simulink model "AutoTransmission"  (R2020a)
settings: Solver=VariableStepAuto  StartTime=0.0  StopTime=10.0  RelTol=1e-3
PostLoadFcn:
  | NE_VEC=[799.9999999999999 1200 1600 2000 2400 2800 3200 3600 4000 4400 4800];
  | TH_VEC=[0;20;30;40;50;60;70;80;90;100];
  | EMAP=[-40 -44 -49 -53 -57 -61 -65 -70 -74 -78 -82;215 117 85 66 44 29 10 -2 -13 -22 -32;245 208 178 148 122 104 85 66 48 33 18;264 260 241 219 193 167 152 133 119 96 85;264 279 282 275 260 238 223 208 189 171 152;267 290 293 297 290 275 260 256 234 212 193;267 297 305 305 305 301 293 282 267 249 226;267 301 308 312 319 323 319 316 297 279 253;267 301 312 319 327 327 327 327 312 293 267;267 301 312 319 327 334 334 334 319 305 275];
  | Iei=0.0219914882835559;
  | CONVERTER_DATA=[0 137.4652089938063 2.232;0.1 137.065019156852 2.075;0.2 135.8644496459891 1.975;0.3 135.6643547275119 1.846;0.4 137.5652564530449 1.72;0.5 140.3665853117251 1.564;0.6 145.2689108144154 1.409;0.7 152.8725177165473 1.254;0.8 162.9773110996437 1.096;0.81 164.2779280697452 1.08;0.82 166.1788297952782 1.061;0.83 167.9796840615726 1.043;0.84 170.0806807055828 1.028;0.85 172.7819621050244 1.012;0.86 175.3831960452274 1.002;0.87 179.5851893332477 1.002;0.88 183.5870877027908 1.001;0.89 189.8900776348212 0.998;0.9 197.6937794554303 0.999;0.92 215.9024170368515 1.001;0.94 244.5159903790849 1.002];
undefined symbols (not defined in the file): Kfactor, speedratio, Torkratio
settings Model: Creator=Hp  LastModifiedBy=Hp

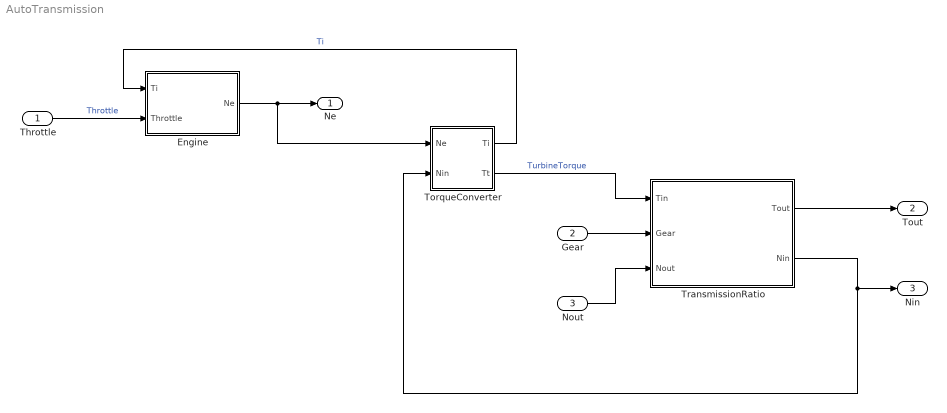
== system AutoTransmission ==
  Throttle : Inport
  Gear : Inport  Port=2
  Nout : Inport  Port=3
  Engine : Subsystem
  TorqueConverter : Subsystem
  TransmissionRatio : Subsystem
  Ne : Outport  Unit=rpm  VectorParamsAs1DForOutWhenUnconnected=off
  Tout : Outport  Port=2
  Nin : Outport  Port=3
  wires:
  TorqueConverter/1(Ti) -> Engine/1(Ti)  "Ti"
  Throttle/1 -> Engine/2(Throttle)  "Throttle"
  Engine/1(Ne) -> TorqueConverter/1(Ne), Ne/1
  TransmissionRatio/2(Nin) -> TorqueConverter/2(Nin), Nin/1
  TorqueConverter/2(Tt) -> TransmissionRatio/1(Tin)  "TurbineTorque"
  Gear/1 -> TransmissionRatio/2(Gear)
  Nout/1 -> TransmissionRatio/3(Nout)
  TransmissionRatio/1(Tout) -> Tout/1

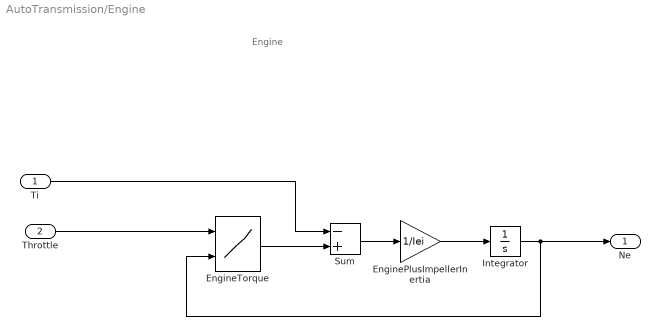
== system AutoTransmission/Engine ==
  note: Engine
  Ti : Inport
  Throttle : Inport  Port=2
  EnginePlusImpellerInertia : Gain  Gain=1/Iei  SaturateOnIntegerOverflow=on  OutDataTypeStr=Inherit: Same as input  ParamDataTypeStr=Inherit: Same as input
  EngineTorque : Lookup_n-D  BreakpointsForDimension1=TH_VEC  BreakpointsForDimension2=NE_VEC  Table=EMAP  InputSameDT=on
  Integrator : Integrator  InitialCondition=1000  LimitOutput=on  UpperSaturationLimit=6000  LowerSaturationLimit=600  ZeroCross=off
  Sum : Sum  Inputs=-+  InputSameDT=on  SaturateOnIntegerOverflow=on  OutDataTypeStr=Inherit: Same as first input
  Ne : Outport
  wires:
  Throttle/1 -> EngineTorque/1
  EnginePlusImpellerInertia/1 -> Integrator/1
  Integrator/1 -> Ne/1, EngineTorque/2
  Sum/1 -> EnginePlusImpellerInertia/1
  Ti/1 -> Sum/1
  EngineTorque/1 -> Sum/2

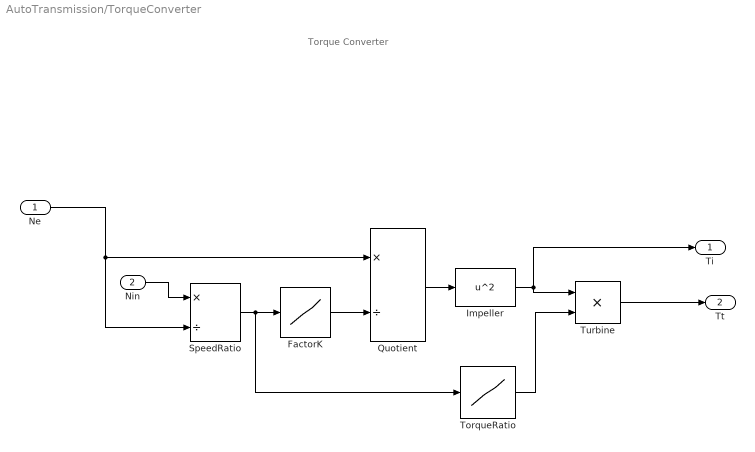
== system AutoTransmission/TorqueConverter ==
  note: Torque Converter
  Ne : Inport
  Nin : Inport  Port=2
  FactorK : Lookup_n-D  NumberOfTableDimensions=1  BreakpointsForDimension1=speedratio  Table=Kfactor  SaturateOnIntegerOverflow=on  InputSameDT=on
  Impeller : Fcn  Expr=u^2
  Quotient : Product  Inputs=*/  InputSameDT=on  SaturateOnIntegerOverflow=on  OutDataTypeStr=Inherit: Same as first input
  SpeedRatio : Product  Inputs=*/  InputSameDT=on  SaturateOnIntegerOverflow=on  OutDataTypeStr=Inherit: Same as first input
  TorqueRatio : Lookup_n-D  NumberOfTableDimensions=1  BreakpointsForDimension1=speedratio  Table=Torkratio  SaturateOnIntegerOverflow=on  InputSameDT=on
  Turbine : Product  InputSameDT=on  SaturateOnIntegerOverflow=on  OutDataTypeStr=Inherit: Same as first input
  Ti : Outport
  Tt : Outport  Port=2
  wires:
  Turbine/1 -> Tt/1
  Ne/1 -> SpeedRatio/2, Quotient/1
  Nin/1 -> SpeedRatio/1
  Impeller/1 -> Ti/1, Turbine/1
  FactorK/1 -> Quotient/2
  SpeedRatio/1 -> FactorK/1, TorqueRatio/1
  Quotient/1 -> Impeller/1
  TorqueRatio/1 -> Turbine/2

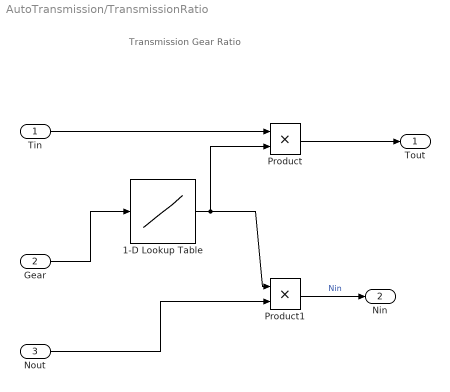
== system AutoTransmission/TransmissionRatio ==
  note: Transmission Gear Ratio
  Tin : Inport
  Gear : Inport  Port=2
  Nout : Inport  Port=3
  1-D Lookup Table : Lookup_n-D  NumberOfTableDimensions=1  BreakpointsForDimension1=[1 2 3 4]  Table=[2.393 1.450 1.000 0.677]  InternalRulePriority=Speed  RndMeth=Simplest  InputSameDT=on
  Product : Product  InputSameDT=on  SaturateOnIntegerOverflow=on  OutDataTypeStr=Inherit: Same as first input
  Product1 : Product  InputSameDT=on  SaturateOnIntegerOverflow=on  OutDataTypeStr=Inherit: Same as first input
  Tout : Outport
  Nin : Outport  Port=2
  wires:
  1-D Lookup Table/1 -> Product1/1, Product/2
  Tin/1 -> Product/1
  Product/1 -> Tout/1
  Product1/1 -> Nin/1  "Nin"
  Gear/1 -> 1-D Lookup Table/1
  Nout/1 -> Product1/2
